simulink model "carmodel_tesla_testing"  (R2018a)
settings: Solver=VariableStepAuto  StartTime=0.0  StopTime=3.8  RelTol=1e-3
settings Model: Creator=abc  LastModifiedBy=abc

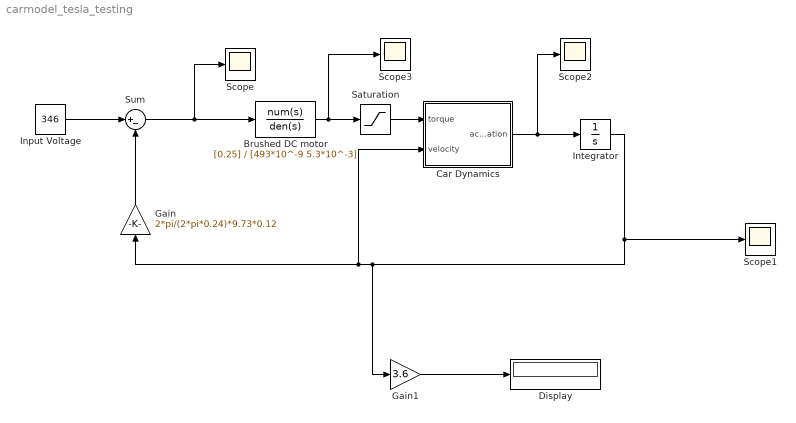
== system carmodel_tesla_testing ==
  Brushed DC motor : TransferFcn  Numerator=[0.25]  Denominator=[493*10^-9 5.3*10^-3]
  Car Dynamics : MATLAB Function  TreatAsAtomicUnit=on
  Display : Display
  Gain : Gain  Gain=2*pi/(2*pi*0.24)*9.73*0.12
  Gain1 : Gain  Gain=3.6
  Input Voltage : Constant  Value=346
  Integrator : Integrator
  Saturation : Saturate  UpperLimit=601  LowerLimit=0
  Scope{,1..3} (4 alike) : Scope
  Sum : Sum  Inputs=|+-
  wires:
  Integrator/1 -> Scope1/1, Gain1/1, Gain/1, Car Dynamics/2(velocity)
  Car Dynamics/1(acceleration) -> Scope2/1, Integrator/1
  Sum/1 -> Scope/1, Brushed DC motor/1
  Gain/1 -> Sum/2
  Input Voltage/1 -> Sum/1
  Brushed DC motor/1 -> Saturation/1, Scope3/1
  Gain1/1 -> Display/1
  Saturation/1 -> Car Dynamics/1(torque)

== matlab function carmodel_tesla_testing/Car Dynamics ==
  data: torque input; acceleration output; velocity input
function acceleration = fn(torque,velocity)
acceleration = (40.5*torque*0.7-413-0.3381*velocity^2)/2108;
